simulink model "testPID"  (R2016b)
settings: Solver=VariableStepAuto  StartTime=0.0  StopTime=5  MaxStep=0.01  RelTol=1e-4  EnableMultiTasking=on
libraries: simulink x1
settings Model: Creator=mihai  LastModifiedBy=mihai
settings DataIOCC: LimitDataPoints=on  SaveOutput=off  SaveTime=off
settings OptimizationCC: ExpressionDepthLimit=2147483647  LifeSpan=1
settings DebuggingCC: UnderspecifiedInitializationDetection=Classic  MergeDetectMultiDrivingBlocksExec=none  FcnCallInpInsideContextMsg=warning  AllowSymbolicDim=off  StateNameClashWarn=warning  SFUnexpectedBacktrackingDiag=warning  SFNoUnconditionalDefaultTransitionDiag=warning  SFExecutionAtInitializationDiag=none
settings GRTTargetCC: TargetLangStandard=C89/C90 (ANSI)  GeneratePreprocessorConditionals=Disable all  CombineOutputUpdateFcns=off  GRTInterface=on

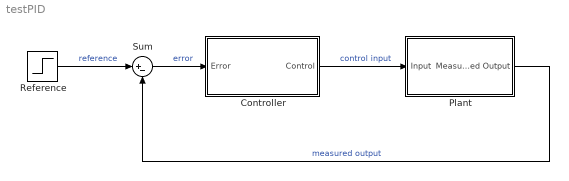
== system testPID ==
  Controller : Subsystem
  Plant : Subsystem
  Reference : Step  SampleTime=0
  Sum : Sum  Inputs=|+-
  wires:
  Reference/1 -> Sum/1  "reference"
  Plant/1(Measured Output) -> Sum/2  "measured output"
  Sum/1 -> Controller/1(Error)  "error"
  Controller/1(Control) -> Plant/1(Input)  "control input"

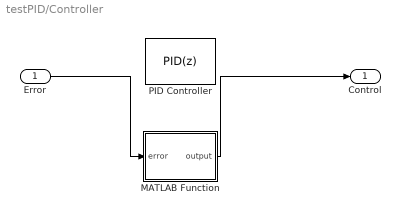
== system testPID/Controller ==
  Error : Inport
  MATLAB Function : MATLAB Function  TreatAsAtomicUnit=on
  PID Controller : simulink/Continuous/PID Controller  Controller=PID  TimeDomain=Discrete-time  SampleTime=0.1  IntegratorMethod=Backward Euler  FilterMethod=Backward Euler  Form=Parallel  UseFilter=on  ControllerParametersSource=internal  P=1.2  I=5  D=0.02  N=20  InitialConditionSource=internal  InitialConditionForIntegrator=0  InitialConditionForFilter=0  ExternalReset=none  LimitOutput=off  UpperSaturationLimit=inf  LowerSaturationLimit=-inf  LinearizeAsGain=on  AntiWindupMode=none  Kb=1  TrackingMode=off  Kt=1  PParamMin=[]  PParamMax=[]  IParamMin=[]  IParamMax=[]  DParamMin=[]  DParamMax=[]  NParamMin=[]  NParamMax=[]  KbParamMin=[]  KbParamMax=[]  KtParamMin=[]  KtParamMax=[]  POutMin=[]  POutMax=[]  IOutMin=[]  IOutMax=[]  DOutMin=[]  DOutMax=[]  NOutMin=[]  NOutMax=[]  KbOutMin=[]  KbOutMax=[]  KtOutMin=[]  KtOutMax=[]  IntegratorOutMin=[]  IntegratorOutMax=[]  FilterOutMin=[]  FilterOutMax=[]  SumOutMin=[]  SumOutMax=[]  SumI1OutMin=[]  SumI1OutMax=[]  SumI2OutMin=[]  SumI2OutMax=[]  SumI3OutMin=[]  SumI3OutMax=[]  SumDOutMin=[]  SumDOutMax=[]  SaturationOutMin=[]  SaturationOutMax=[]  IntegratorContinuousStateAttributes=''  IntegratorStateMustResolveToSignalObject=off  IntegratorRTWStateStorageClass=Auto  FilterContinuousStateAttributes=''  FilterStateMustResolveToSignalObject=off  FilterRTWStateStorageClass=Auto  DifferentiatorICPrevScaledInput=0  DifferentiatorOutMin=[]  DifferentiatorOutMax=[]
  Control : Outport
  wires:
  Error/1 -> MATLAB Function/1(error)
  MATLAB Function/1(output) -> Control/1

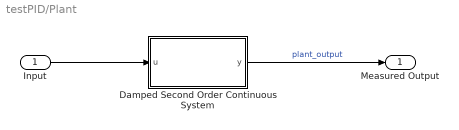
== system testPID/Plant ==
  Input : Inport
  Damped Second Order Continuous System : Subsystem  mask{wn=16, zeta=0.6}
      mask prompts: wn "Undamped natural frequency (wn, rad/s)"; zeta "Damping factor (zeta)"
  Measured Output : Outport
  wires:
  Input/1 -> Damped Second Order Continuous System/1(u)
  Damped Second Order Continuous System/1(y) -> Measured Output/1  "plant_output"

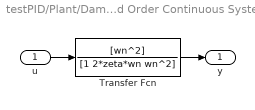
== system testPID/Plant/Damped Second Order Continuous System ==
  u : Inport
  Transfer Fcn : TransferFcn  Numerator=[wn^2]  Denominator=[1 2*zeta*wn wn^2]
  y : Outport
  wires:
  Transfer Fcn/1 -> y/1
  u/1 -> Transfer Fcn/1

== matlab function testPID/Controller/MATLAB Function ==
  data: error input; output output
function output = fcn(error)
%controller for the multi agent formation control. PID. Inputs should
%controllerOutput is the speed for each Sphero
persistent previousError integral;
if isempty(previousError)
    previousError = 0;
end

if isempty(integral)
    integral = 0;
end
% 
% Kp = PIDGains(1);
% Ki = PIDGains(2);
% Kd = PIDGains(3);

% N = 20;
% Ts = 0.1;
dt = 0.1;
Kp = 2.5;
Ki = 0.1;
Kd = 0;

%actual control
saturation = 10;
integral = integral + error*dt;
integral = min(saturation, max(-saturation, integral));
derivative = (error - previousError) ./ dt;

output = Kp * error + Ki * integral + Kd * derivative;

%saturation
%output = min(0.4, max(0, output));

previousError = error;

end
